simulink model "ModeloSyncGen"  (R2014a)
settings: Solver=ode45  StartTime=0.0  StopTime=10.0  RelTol=1e-3
values from neighbouring files (symbols this model uses):
  I = S/V    (= 18500)    [CalcSteady1.m]    (also in Main.m = (H*S)/(0.5*W.^2); Main2.m = (H*S)/(0.5*W.^2); SolverODE.m = inv(L)*lambda_vec)
  Ld = 7e-3    (= 0.007)    [CalcSteady1.m]    (also in CalcSteady2.m; Main.m; Main2.m; SolverODE.m)
  Lf = 7.384e-3    (= 0.007384)    [CalcSteady1.m]    (also in CalcSteady2.m; Main.m; Main2.m; SolverODE.m)
  Lm = 6.656e-3    (= 0.006656)    [CalcSteady1.m]    (also in CalcSteady2.m; Main.m; Main2.m; SolverODE.m)
  Lq = 5.61e-3    (= 0.00561)    [CalcSteady1.m]    (also in CalcSteady2.m; Main.m; Main2.m; SolverODE.m)
  Rf = 0.985e-3    (= 0.000985)    [CalcSteady1.m]    (also in CalcSteady2.m; Main.m; Main2.m; SolverODE.m)
  Rs = 1.6e-3    (= 0.0016)    [CalcSteady1.m]    (also in CalcSteady2.m; Main.m; Main2.m; SolverODE.m)
  ws = 2*pi*50    (= 314.159265359)    [CalcSteady1.m]    (also in CalcSteady2.m; Main.m; Main2.m; SolverODE.m)
libraries: dspinverses x1
settings Model: Creator=Eduardo  LastModifiedBy=Eduardo

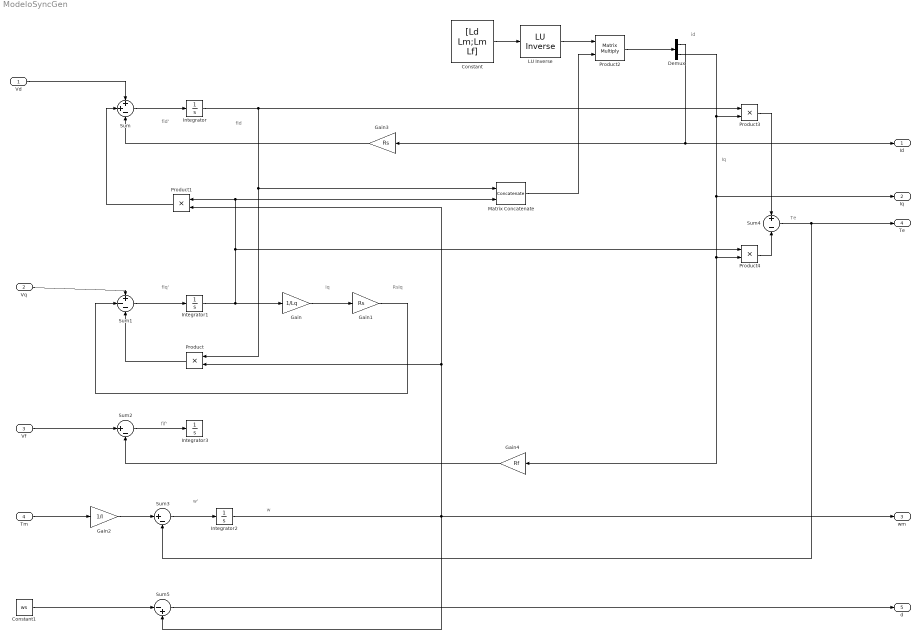
== system ModeloSyncGen ==
  note: Te
  note: fif'
  note: Iq
  note: id
  note: w
  note: w'
  note: RsIq
  note: iq
  note: fiq'
  note: fid
  note: fid'
  Vd : Inport
  Vq : Inport  Port=2
  Vf : Inport  Port=3
  Tm : Inport  Port=4
  " LU Inverse" : dspinverses/ LU Inverse
  Constant : Constant  Value=[Ld Lm;Lm Lf]
  Constant1 : Constant  Value=ws
  Demux : Demux  Outputs=2
  Gain : Gain  Gain=1/Lq
  Gain1 : Gain  Gain=Rs
  Gain2 : Gain  Gain=1/I
  Gain3 : Gain  Gain=Rs
  Gain4 : Gain  Gain=Rf
  Integrator{,1..3} (4 alike) : Integrator
  Matrix Concatenate : Concatenate  Mode=Multidimensional array  ConcatenateDimension=2
  Product{,1,3..4} (4 alike) : Product
  Product2 : Product  Multiplication=Matrix(*)
  Sum : Sum  Inputs=++-
  Sum1 : Sum  Inputs=+--
  Sum2 : Sum  Inputs=|+-
  Sum3 : Sum  Inputs=|+-
  Sum4 : Sum  Inputs=+|-
  Sum5 : Sum  Inputs=|-+
  Id : Outport
  "Iq " : Outport  Port=2
  wm : Outport  Port=3
  Te : Outport  Port=4
  d : Outport  Port=5
  wires:
  Vd/1 -> Sum/1
  Vq/1 -> Sum1/1
  Vf/1 -> Sum2/1
  Sum/1 -> Integrator/1
  Product/1 -> Sum1/3
  Integrator/1 -> Product/1, Matrix Concatenate/1, Product3/1
  Sum1/1 -> Integrator1/1
  Integrator1/1 -> Product4/1, Matrix Concatenate/2, Product1/1, Gain/1
  Gain/1 -> Gain1/1
  Gain1/1 -> Sum1/2
  Tm/1 -> Gain2/1
  Gain2/1 -> Sum3/1
  Sum3/1 -> Integrator2/1
  Integrator2/1 -> Sum5/2, Product/2, Product1/2, wm/1
  Constant/1 -> " LU Inverse"/1
  " LU Inverse"/1 -> Product2/1
  Matrix Concatenate/1 -> Product2/2
  Product2/1 -> Demux/1
  Demux/1 -> Id/1, Gain3/1
  Product1/1 -> Sum/2
  Gain3/1 -> Sum/3
  Demux/2 -> Gain4/1, Product4/2, "Iq "/1, Product3/2
  Gain4/1 -> Sum2/2
  Sum2/1 -> Integrator3/1
  Product3/1 -> Sum4/1
  Product4/1 -> Sum4/2
  Sum4/1 -> Sum3/2, Te/1
  Constant1/1 -> Sum5/1
  Sum5/1 -> d/1
